simulink model "AWES3_CL_wTether_v4_PM"  (R2022a)
settings: Solver=ode3  StartTime=0  StopTime=simInit.TSIM  FixedStep=simInit.dt  RelTol=1e-3
values from neighbouring files (symbols this model uses):
  complex_tether_flag = 1    [run_sim.m]
  Ft_max = 1870    [run_sim.m]
  q = 0    [barrier_optimization.m]
  r = 0    [barrier_optimization.m]
  random_seed = [ 24335       17059       17670        1747]    [run_sim.m]
  safety_controller = false    [run_sim.m]
  turbulence = true    [run_sim.m]
undefined symbols (not defined in the file or in its folder): aeroModel, alpha_max, alpha_min, alpha_options, base_windspeed, constr, DiscIntNeverNeededParam, dx, ENVMT, F, grid_max, grid_min, HDBK, I_table, Light, MIL, mu_max, mu_min, mu_options, P_AP2, params, SampleTime, simInit, T, u0_sim, winchParameter, x0_sim
libraries: simulink x30, aerolibwind2 x14, dspstat3 x2, pid_lib x1, aerolibwindfilters x1, aerolibcommonsys x1, matrix_library x1
(part 1 of 5)
settings Model: SimulationMode=accelerator  ExtModeTrigDuration=100  Creator=Sebastian  LastModifiedBy=kebl6571
settings SolverCC: AlgebraicLoopSolver=LineSearch  DecoupledContinuousIntegration=on  MinimalZcImpactIntegration=on
settings DataIOCC: SaveFormat=StructureWithTime  SaveOutput=off  DSMLogging=off  SaveTime=off  StateSaveName=tmp_raccel_xout  OutputSaveName=logged_signals  SignalLoggingName=logged_signals  LoggingToFile=on  LoggingFileName=log.mat
settings OptimizationCC: BufferReuse=off  GlobalBufferReuse=off  ExpressionFolding=off  LocalBlockOutputs=off  EfficientMapNaN2IntZero=off  LifeSpan=inf  OptimizeDataStoreBuffers=off  BusAssignmentInplaceUpdate=off
settings DebuggingCC: ReadBeforeWriteMsg=DisableAll  WriteAfterWriteMsg=DisableAll  WriteAfterReadMsg=DisableAll  ArtificialAlgebraicLoopMsg=none  SaveWithDisabledLinksMsg=none  SaveWithParameterizedLinksMsg=none  MaskedZcDiagnostic=none  IgnoredZcDiagnostic=none  InheritedTsInSrcMsg=none  MultiTaskDSMMsg=none  TasksWithSamePriorityMsg=none  SigSpecEnsureSampleTimeMsg=none  BusObjectLabelMismatch=none  RootOutportRequireBusObject=none  AllowSymbolicDim=off  UnknownTsInhSupMsg=none  ModelReferenceDataLoggingMessage=none  ModelReferenceSymbolNameMessage=none  OperatingPointInterfaceChecksumMismatchMsg=none  InitInArrayFormatMsg=none  SFUnusedDataAndEventsDiag=none  SFUnexpectedBacktrackingDiag=none  SFInvalidInputDataAccessInChartInitDiag=none  SFNoUnconditionalDefaultTransitionDiag=none  SFTransitionOutsideNaturalParentDiag=none  SFUnreachableExecutionPathDiag=none  SFUndirectedBroadcastEventsDiag=none  SFTransitionActionBeforeConditionDiag=none  SFTemporalDelaySmallerThanSampleTimeDiag=none  SFSelfTransitionDiag=none  SFExecutionAtInitializationDiag=none  SFMachineParentedDataDiag=none  UnitsInconsistencyMsg=none  ArithmeticOperatorsInVariantConditions=warning
settings HardwareCC: TargetBitPerPointer=64  TargetBitPerSizeT=64  TargetBitPerPtrDiffT=64  TargetLongLongMode=on  TargetIntDivRoundTo=Zero  TargetEndianess=LittleEndian  TargetWordSize=64  TargetHWDeviceType=MATLAB Host  ProdEqTarget=off
settings ModelReferenceCC: UpdateModelReferenceTargets=IfOutOfDate  PropagateSignalLabelsOutOfModel=off
settings SFSimCC: SFSimEcho=off  SimUseLocalCustomCode=off  CustomCodeUndefinedFunction=UseInterfaceOnly
settings RTWCC: DLArmComputeVersion=19.05
settings CodeAppCC: MaxIdLength=128
settings GRTTargetCC: TargetLangStandard=C89/C90 (ANSI)  CombineOutputUpdateFcns=off  GRTInterface=on
settings ConfigComp: CovMetricSettings=dw  CovSaveCumulativeToWorkspaceVar=on  CovSaveSingleToWorkspaceVar=on  CovExternalEMLEnable=off

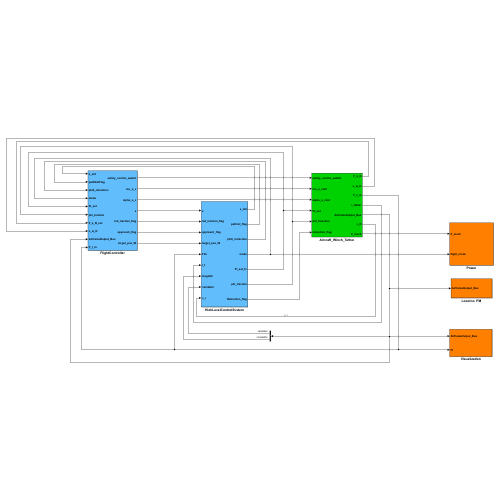
[thumbnail: Simulink's stored preview of the top-level diagram]
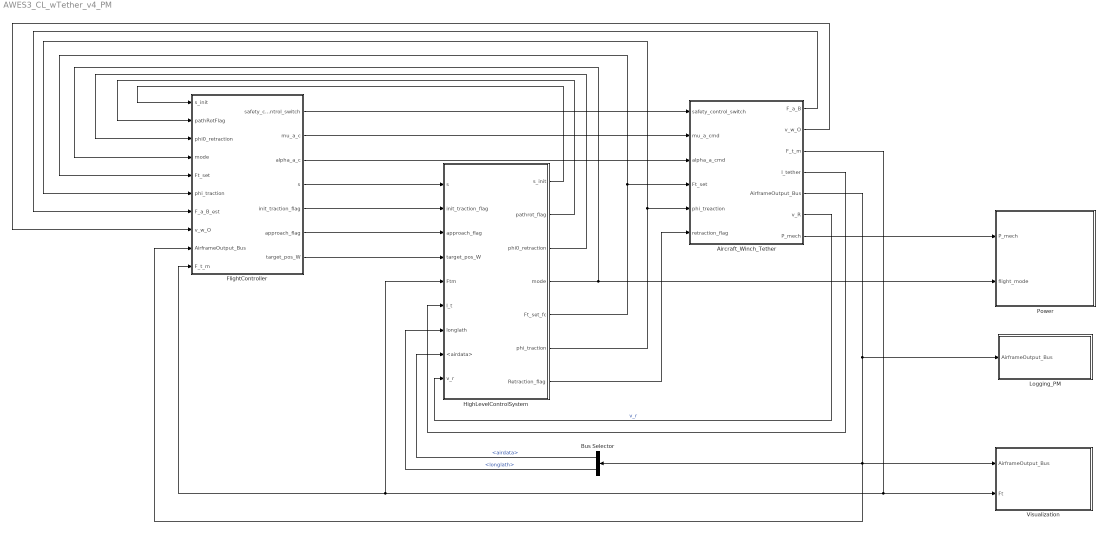
== system AWES3_CL_wTether_v4_PM ==
  Aircraft_Winch_Tether : Subsystem
  Bus Selector : BusSelector  OutputSignals=airdata,longlath
  FlightController : Subsystem
  HighLevelControlSystem : Subsystem
  Logging_PM : Subsystem  mask{logging_ts=0.01}
  Power : Subsystem  mask{sample_time=simInit.Ts_power_conv_check, min_cycles=4}
  Visualization : Subsystem
  wires:
  Aircraft_Winch_Tether/4(l_tether) -> HighLevelControlSystem/6(l_t)
  Aircraft_Winch_Tether/3(F_t_m) -> HighLevelControlSystem/5(Ftm), FlightController/10(F_t_m), Visualization/2(Ft)
  Aircraft_Winch_Tether/5(AirframeOutput_Bus) -> Visualization/1(AirframeOutput_Bus), FlightController/9(AirframeOutput_Bus), Bus Selector/1, Logging_PM/1(AirframeOutput_Bus)
  Bus Selector/2 -> HighLevelControlSystem/7(longlath)  "<longlath>"
  Aircraft_Winch_Tether/1(F_a_B) -> FlightController/7(F_a_B_est)
  Aircraft_Winch_Tether/2(v_w_O) -> FlightController/8(v_w_O)
  HighLevelControlSystem/4(mode) -> FlightController/4(mode), Power/2(flight_mode)
  HighLevelControlSystem/3(phi0_retraction) -> FlightController/3(phi0_retraction)
  HighLevelControlSystem/2(pathrot_flag) -> FlightController/2(pathRotFlag)
  HighLevelControlSystem/1(s_init) -> FlightController/1(s_init)
  HighLevelControlSystem/6(phi_traction) -> Aircraft_Winch_Tether/5(phi_treaction), FlightController/6(phi_traction)
  FlightController/4(s) -> HighLevelControlSystem/1(s)
  FlightController/5(init_traction_flag) -> HighLevelControlSystem/2(init_traction_flag)
  FlightController/6(approach_flag) -> HighLevelControlSystem/3(approach_flag)
  FlightController/7(target_pos_W) -> HighLevelControlSystem/4(target_pos_W)
  HighLevelControlSystem/5(Ft_set_fc) -> Aircraft_Winch_Tether/4(Ft_set), FlightController/5(Ft_set)
  HighLevelControlSystem/7(Retraction_flag) -> Aircraft_Winch_Tether/6(retraction_flag)
  Aircraft_Winch_Tether/6(v_R) -> HighLevelControlSystem/9(v_r)  "v_r"
  Bus Selector/1 -> HighLevelControlSystem/8(<airdata>)  "<airdata>"
  FlightController/3(alpha_a_c) -> Aircraft_Winch_Tether/3(alpha_a_cmd)
  FlightController/2(mu_a_c) -> Aircraft_Winch_Tether/2(mu_a_cmd)
  FlightController/1(safety_control_switch) -> Aircraft_Winch_Tether/1(safety_control_switch)
  Aircraft_Winch_Tether/7(P_mech) -> Power/1(P_mech)

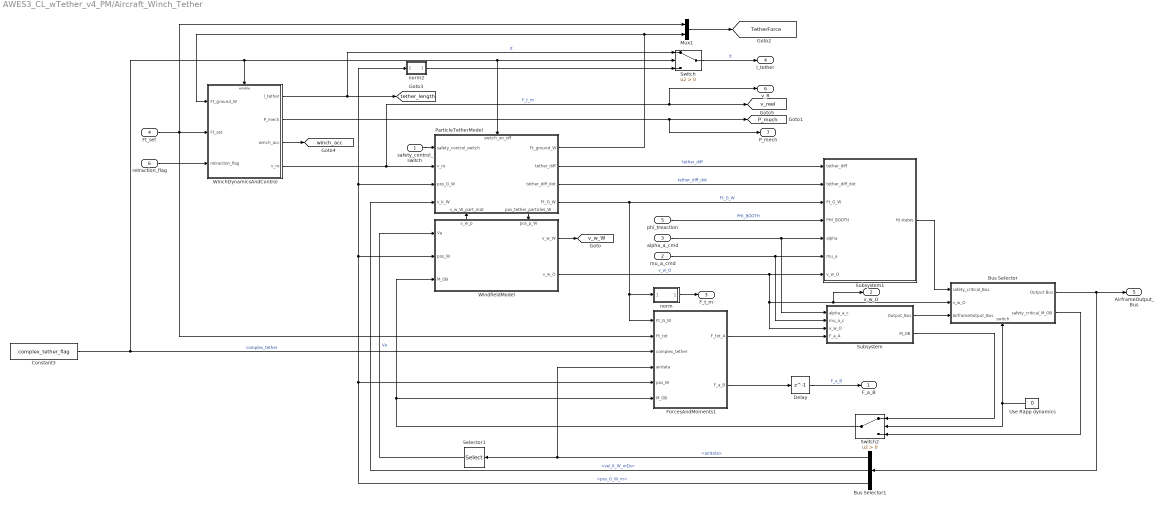
== system AWES3_CL_wTether_v4_PM/Aircraft_Winch_Tether ==
  safety_control_switch : Inport
  mu_a_cmd : Inport  Port=2  PortDimensions=1
  alpha_a_cmd : Inport  Port=3  PortDimensions=1
  Ft_set : Inport  Port=4  PortDimensions=1
  phi_treaction : Inport  Port=5  PortDimensions=1
  retraction_flag : Inport  Port=6  PortDimensions=1
  Bus Selector1 : BusSelector  OutputSignals=airdata,vel_K_W_mDs,pos_G_W_m
  Bus Selector : Subsystem
      settings: PortSchema="{\"entries\":[{\"content\":{\"sides\":[{\"content\":{\"connectorIds\":[\"In1\",\"In2\",\"In3\"]},\"type\":\"ConnectorPlacement.EquallySpacedRectSide\",\"uuid\":\"e2ab3ba8-f9f5-4bb0-af4c-3fe158d9c7f2\"},{\"content\":{\"connectorIds\":[\"Out1\",\"Out2\"],\"side\":\"RIGHT\"},\"type\":\"ConnectorPlacement.EquallySpacedRectSide\",\"uuid\":\"54795f1d-c357-49f1-9330-7dd1b9d78901\"},{\"content\":{\"connectorIds\":[],\"side\":\"TOP\"},\"type\":\"ConnectorPlacement.EquallySpacedRectSide\",\"uuid\":\"9cb9c5b8-3137-45d1-bfe3-c0a6ae4a4824\"},{\"content\":{\"connectorIds\":[\"In4\"],\"side\":\"BOTTOM\"},\"type\":\"ConnectorPlacement.EquallySpacedRectSide\",\"uuid\":\"b9adb0a8-6fab-4e9c-b487-f47b7669de1a\"}]},\"type\":\"ConnectorPlacement.EquallySpacedConnector\",\"uuid\":\"c66c7c14-26bf-43dc-ba87-485e61b07403\"}],\"packageUris\":[\"http://schema.mathworks.com/mf0/Connector/R2020b\"],\"version\":\"1.0\"}"
  Constant3 : Constant  Value=complex_tether_flag
  Delay : Delay  DelayLength=1  InitialCondition=[1;1;-P_AP2.mass*10]
  ForcesAndMoments1 : Subsystem
  Mux1 : Mux  Inputs=2
  ParticleTetherModel : Subsystem
      settings: PortSchema="{\"entries\":[{\"content\":{\"sides\":[{\"content\":{\"connectorIds\":[\"In1\",\"In2\",\"In3\",\"In4\"]},\"type\":\"ConnectorPlacement.EquallySpacedRectSide\",\"uuid\":\"ca78405c-c6d3-477d-b0a8-668910473732\"},{\"content\":{\"connectorIds\":[\"Out1\",\"Out2\",\"Out3\",\"Out4\"],\"side\":\"RIGHT\"},\"type\":\"ConnectorPlacement.EquallySpacedRectSide\",\"uuid\":\"a5c38c1a-07d2-4efb-bc49-b1eee8e8eb74\"},{\"content\":{\"connectorIds\":[\"In5\"],\"side\":\"TOP\"},\"type\":\"ConnectorPlacement.EquallySpacedRectSide\",\"uuid\":\"403c634d-ac4b-4d6b-b076-489af818e83e\"},{\"content\":{\"connectorIds\":[\"In6\",\"Out5\"],\"side\":\"BOTTOM\"},\"type\":\"ConnectorPlacement.EquallySpacedRectSide\",\"uuid\":\"4ef9c4e3-0026-4b23-9119-1a1dd44b231c\"}]},\"type\":\"ConnectorPlacement.EquallySpacedConnector\",\"uuid\":\"599465da-399f-49af-adc9-4f96ef4c12cd\"}],\"packageUris\":[\"http://schema.mathworks.com/mf0/Connector/R2020b\"],\"version\":\"1.0\"}"
  Selector1 : Selector  InputPortWidth=3  IndexOptions=Index vector (dialog)  Indices=1  OutputSizes=1
  Subsystem : Subsystem
      settings: MinAlgLoopOccurrences=on
  Subsystem1 : Subsystem
      settings: MinAlgLoopOccurrences=on
  Switch : Switch  Criteria=u2 > Threshold  SaturateOnIntegerOverflow=off  InputSameDT=off
  Switch2 : Switch  Criteria=u2 > Threshold  SaturateOnIntegerOverflow=off  InputSameDT=off
  Use Rapp dynamics : Constant  Value=0
  "WinchDynamicsAndControl " : Subsystem
  WindfieldModel : Subsystem  TreatAsAtomicUnit=on
      settings: MinAlgLoopOccurrences=on  PortSchema="{\"entries\":[{\"content\":{\"sides\":[{\"content\":{\"connectorIds\":[\"In1\",\"In2\",\"In3\"]},\"type\":\"ConnectorPlacement.EquallySpacedRectSide\",\"uuid\":\"5214d961-fdb0-4544-8128-59e00c6649fb\"},{\"content\":{\"connectorIds\":[\"Out1\",\"Out2\"],\"side\":\"RIGHT\"},\"type\":\"ConnectorPlacement.EquallySpacedRectSide\",\"uuid\":\"cdd5f5d4-5bc0-4393-ba09-7e71cbb012db\"},{\"content\":{\"connectorIds\":[\"Out3\",\"In4\"],\"side\":\"TOP\"},\"type\":\"ConnectorPlacement.EquallySpacedRectSide\",\"uuid\":\"608e5071-fd31-4d22-8974-ba91486c9a41\"}]},\"type\":\"ConnectorPlacement.EquallySpacedConnector\",\"uuid\":\"a45b9672-4292-4679-90b4-f0e0bc01633b\"}],\"packageUris\":[\"http://schema.mathworks.com/mf0/Connector/R2020b\"],\"version\":\"1.0\"}"
  norm : Subsystem
  norm2 : Subsystem
  F_a_B : Outport  VectorParamsAs1DForOutWhenUnconnected=off
  v_w_O : Outport  Port=2  VectorParamsAs1DForOutWhenUnconnected=off
  F_t_m : Outport  Port=3  VectorParamsAs1DForOutWhenUnconnected=off
  l_tether : Outport  Port=4  VectorParamsAs1DForOutWhenUnconnected=off
  AirframeOutput_Bus : Outport  Port=5  VectorParamsAs1DForOutWhenUnconnected=off
  v_R : Outport  Port=6  VectorParamsAs1DForOutWhenUnconnected=off
  P_mech : Outport  Port=7  VectorParamsAs1DForOutWhenUnconnected=off
  tag scope: P_mech=global, TetherForce=global, tether_length=global, v_reel=global, v_w_W=global, winch_acc=global
  wires:
  ForcesAndMoments1/2(F_a_B) -> Delay/1
  WindfieldModel/1(v_w_W) -> [v_w_W]
  WindfieldModel/3(v_w_p) -> ParticleTetherModel/6(v_w_W_part_mat)
  ParticleTetherModel/1(Ft_ground_W) -> Mux1/2, "WinchDynamicsAndControl "/1(Ft_ground_W)
  Ft_set/1 -> "WinchDynamicsAndControl "/2(Ft_set), Mux1/1, ForcesAndMoments1/2(Ft_tot)
  ParticleTetherModel/5(pos_tether_particles_W) -> WindfieldModel/4(pos_p_W)
  Delay/1 -> F_a_B/1  "F_a_B"
  WindfieldModel/2(v_w_O) -> Bus Selector/2(v_w_O), v_w_O/1, Subsystem/3(v_w_O), Subsystem1/7(v_w_O)  "v_w_O"
  Switch/1 -> l_tether/1  "lt"
  ParticleTetherModel/4(Ft_G_W) -> norm/1(Ft_G_W), ForcesAndMoments1/1(Ft_G_W), Subsystem1/3(Ft_G_W)  "Ft_G_W"
  "WinchDynamicsAndControl "/4(v_ro) -> ParticleTetherModel/2(v_ro), v_R/1, [v_reel]  "F_t_m"
  Constant3/1 -> ParticleTetherModel/5(switch_on_off), Switch/2, "WinchDynamicsAndControl "/Enable, ForcesAndMoments1/3(complex_tether)  "complex_tether"
  mu_a_cmd/1 -> Subsystem/2(mu_a_c), Subsystem1/6(mu_a)
  Switch2/1 -> ForcesAndMoments1/6(M_OB), WindfieldModel/3(M_OB)
  "WinchDynamicsAndControl "/3(winch_acc) -> [winch_acc]
  "WinchDynamicsAndControl "/2(P_mech) -> P_mech/1, [P_mech]
  Mux1/1 -> [TetherForce]
  "WinchDynamicsAndControl "/1(l_tether) -> [tether_length], Switch/1  "lt"
  alpha_a_cmd/1 -> Subsystem/1(alpha_a_c), Subsystem1/5(alpha)
  Bus Selector1/2 -> ParticleTetherModel/4(v_k_W)  "<vel_K_W_mDs>"
  Bus Selector1/3 -> ForcesAndMoments1/5(pos_W), ParticleTetherModel/3(pos_G_W), norm2/1(<pos_G_W_m>), WindfieldModel/2(pos_W)  "<pos_G_W_m>"
  Bus Selector/2(safety_critical_M_OB) -> Switch2/3
  Bus Selector1/1 -> Selector1/1, ForcesAndMoments1/4(airdata)  "<airdata>"
  Selector1/1 -> WindfieldModel/1(Va)  "Va"
  Use Rapp dynamics/1 -> Switch2/2, Bus Selector/4(switch)
  retraction_flag/1 -> "WinchDynamicsAndControl "/3(retraction_flag)
  safety_control_switch/1 -> ParticleTetherModel/1(safety_control_switch)
  Subsystem1/1(HJ states) -> Bus Selector/1(safety_critical_Bus)
  ParticleTetherModel/2(tether_diff) -> Subsystem1/1(tether_diff)  "tether_diff"
  ParticleTetherModel/3(tether_diff_dot) -> Subsystem1/2(tether_diff_dot)  "tether_diff_dot"
  phi_treaction/1 -> Subsystem1/4(PHI_BOOTH)  "PHI_BOOTH"
  ForcesAndMoments1/1(F_tot_A) -> Subsystem/4(F_a_A)
  Subsystem/2(M_OB) -> Switch2/1
  Subsystem/1(Output_Bus) -> Bus Selector/3(AirframeOutput_Bus)
  norm/1(F_t_m) -> F_t_m/1
  norm2/1(Out1) -> Switch/3
  Bus Selector/1(Output Bus) -> Bus Selector1/1, AirframeOutput_Bus/1

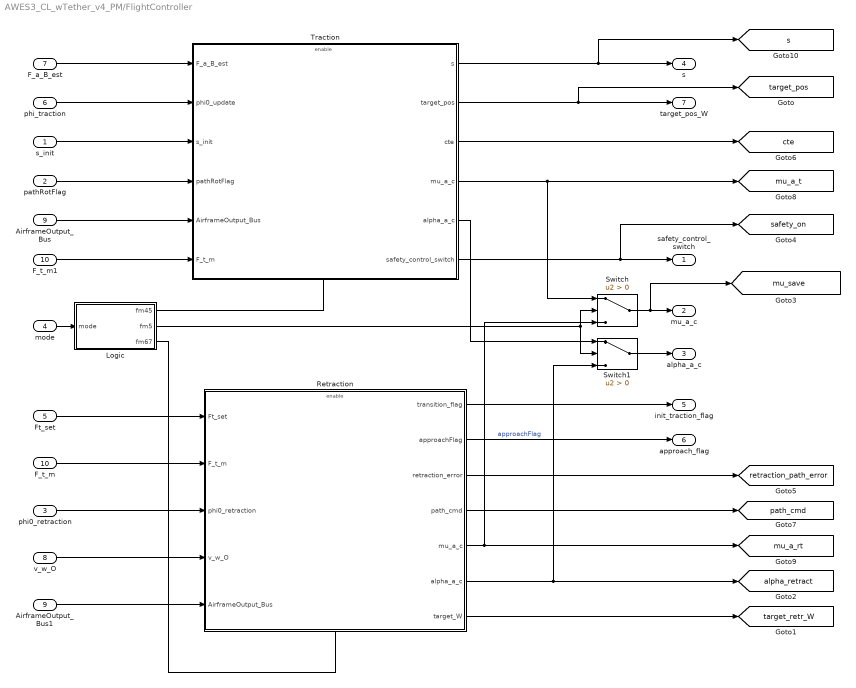
== system AWES3_CL_wTether_v4_PM/FlightController ==
  s_init : Inport
  pathRotFlag : Inport  Port=2
  phi0_retraction : Inport  Port=3
  mode : Inport  Port=4
  Ft_set : Inport  Port=5
  phi_traction : Inport  Port=6
  F_a_B_est : Inport  Port=7
  v_w_O : Inport  Port=8
  AirframeOutput_Bus : Inport  Port=9
  F_t_m : Inport  Port=10
  AirframeOutput_Bus1 : InportShadow  Port=9
  F_t_m1 : InportShadow  Port=10
  Logic : Subsystem
  Retraction : Subsystem
  Switch : Switch  Criteria=u2 > Threshold  SaturateOnIntegerOverflow=off  InputSameDT=off
  Switch1 : Switch  Criteria=u2 > Threshold  SaturateOnIntegerOverflow=off  InputSameDT=off
  Traction : Subsystem
  safety_control_switch : Outport
  mu_a_c : Outport  Port=2  VectorParamsAs1DForOutWhenUnconnected=off
  alpha_a_c : Outport  Port=3  VectorParamsAs1DForOutWhenUnconnected=off
  s : Outport  Port=4  VectorParamsAs1DForOutWhenUnconnected=off
  init_traction_flag : Outport  Port=5  VectorParamsAs1DForOutWhenUnconnected=off
  approach_flag : Outport  Port=6  VectorParamsAs1DForOutWhenUnconnected=off
  target_pos_W : Outport  Port=7  VectorParamsAs1DForOutWhenUnconnected=off
  tag scope: alpha_retract=global, cte=global, mu_a_rt=global, mu_a_t=global, mu_save=global, path_cmd=global, retraction_path_error=global, s=global, safety_on=global, target_pos=global, target_retr_W=global
  wires:
  F_a_B_est/1 -> Traction/1(F_a_B_est)
  phi_traction/1 -> Traction/2(phi0_update)
  s_init/1 -> Traction/3(s_init)
  pathRotFlag/1 -> Traction/4(pathRotFlag)
  Ft_set/1 -> Retraction/1(Ft_set)
  F_t_m/1 -> Retraction/2(F_t_m)
  phi0_retraction/1 -> Retraction/3(phi0_retraction)
  v_w_O/1 -> Retraction/4(v_w_O)
  mode/1 -> Logic/1(mode)
  Logic/1(fm45) -> Traction/Enable
  Logic/2(fm5) -> Switch1/2, Switch/2
  Logic/3(fm67) -> Retraction/Enable
  Retraction/5(mu_a_c) -> [mu_a_rt], Switch/3
  Switch/1 -> [mu_save], mu_a_c/1
  Retraction/1(transition_flag) -> init_traction_flag/1
  Retraction/2(approachFlag) -> approach_flag/1  "approachFlag"
  Traction/2(target_pos) -> [target_pos], target_pos_W/1
  Traction/1(s) -> s/1, [s]
  AirframeOutput_Bus/1 -> Traction/5(AirframeOutput_Bus)
  AirframeOutput_Bus1/1 -> Retraction/5(AirframeOutput_Bus)
  Retraction/6(alpha_a_c) -> Switch1/3, [alpha_retract]
  Retraction/3(retraction_error) -> [retraction_path_error]
  Traction/3(cte) -> [cte]
  Retraction/4(path_cmd) -> [path_cmd]
  Traction/4(mu_a_c) -> Switch/1, [mu_a_t]
  Switch1/1 -> alpha_a_c/1
  Traction/5(alpha_a_c) -> Switch1/1
  Retraction/7(target_W) -> [target_retr_W]
  Traction/6(safety_control_switch) -> [safety_on], safety_control_switch/1
  F_t_m1/1 -> Traction/6(F_t_m)

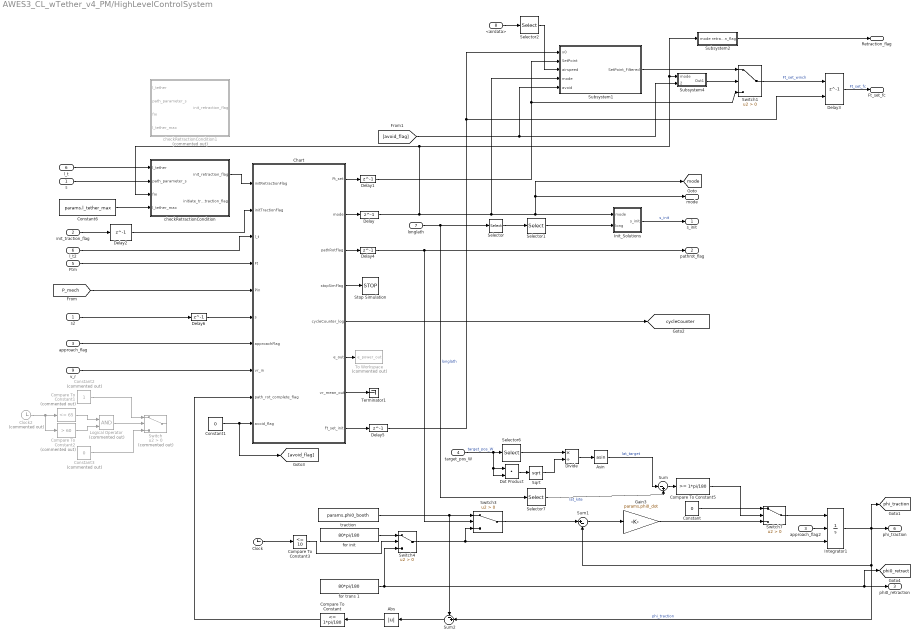
== system AWES3_CL_wTether_v4_PM/HighLevelControlSystem ==
  s : Inport
  init_traction_flag : Inport  Port=2
  approach_flag : Inport  Port=3
  target_pos_W : Inport  Port=4
  Ftm : Inport  Port=5
  l_t : Inport  Port=6
  longlath : Inport  Port=7
  <airdata> : Inport  Port=8
  v_r : Inport  Port=9
  Abs : Abs  SaturateOnIntegerOverflow=off
  Asin : Trigonometry  Operator=asin
  Chart : Stateflow chart  TreatAsAtomicUnit=on  mask{Ft_set_traction=params.Ft_set_traction, Ft_set_traction_low=params.Ft_set_traction_low, Ft_set_retraction=params.Ft_set_retraction, l_t_min_max=params.l_t_min_max, cycleCounterMin=3, cycleCounterMax=5, e_conv=constr.F_t_max*constr.winchParameter.v_max*0.001, Vamin=constr.vamin, vr_mean_min=params.vr_mean_min, Ft_set_avoidance=1200, trac_count_max=10}
  Clock : Clock
  Clock2 : Clock  Commented=on
  Compare To Constant : simulink/Logic and Bit Operations/Compare To Constant  relop=<=  const=1*pi/180  OutDataTypeStr=boolean
  Compare To Constant1 : simulink/Logic and Bit Operations/Compare To Constant  Commented=on  relop=<=  const=65  OutDataTypeStr=boolean
  Compare To Constant2 : simulink/Logic and Bit Operations/Compare To Constant  Commented=on  relop=>  const=60  OutDataTypeStr=boolean
  Compare To Constant3 : simulink/Logic and Bit Operations/Compare To Constant  relop=<=  const=10  OutDataTypeStr=boolean
  Compare To Constant5 : simulink/Logic and Bit Operations/Compare To Constant  relop=>=  const=1*pi/180  OutDataTypeStr=boolean
  Constant : Constant  Value=0
  Constant1 : Constant  Value=0
  Constant2 : Constant  Commented=on
  Constant3 : Constant  Commented=on  Value=0
  Constant6 : Constant  Value=params.l_tether_max
  Delay : Delay  DelayLength=1  InitialCondition=5
  Delay1 : Delay  DelayLength=1  InitialCondition=100
  Delay2 : Delay  DelayLength=1  InitialCondition=5
  Delay3 : Delay  DelayLength=1  InitialConditionSource=Input port  InitialCondition=500
      settings: InputPortMap=u0,p4
  Delay4 : Delay  DelayLength=1
  Delay5 : Delay  DelayLength=1  InitialCondition=1000
  Delay6 : Delay  DelayLength=1  InitialCondition=0
  Divide : Product  Inputs=*/
  Dot Product : DotProduct  OutDataTypeStr=Inherit: Inherit via internal rule
  Gain3 : Gain  Gain=params.phi0_dot
  Init_Solutions : Stateflow chart  TreatAsAtomicUnit=on
  Integrator1 : Integrator  ExternalReset=rising  InitialConditionSource=external
  Logical Operator : Logic  Commented=on  AllPortsSameDT=off  OutDataTypeStr=boolean
  Selector : Selector  InputPortWidth=3  IndexOptions=Index vector (dialog)  Indices=1:2  OutputSizes=1
  Selector1 : Selector  InputPortWidth=2  IndexOptions=Index vector (dialog)  Indices=1  OutputSizes=1
  Selector2 : Selector  InputPortWidth=3  IndexOptions=Index vector (dialog)  Indices=1  OutputSizes=1
  Selector6 : Selector  InputPortWidth=3  IndexOptions=Index vector (dialog)  Indices=3  OutputSizes=1
  Selector7 : Selector  InputPortWidth=3  IndexOptions=Index vector (dialog)  Indices=2  OutputSizes=1
  Sqrt : Sqrt
  Stop Simulation : Stop
  Subsystem1 : Subsystem  mask{w0=0.25}
  Subsystem2 : Subsystem
  Subsystem4 : Subsystem
  Sum : Sum  Inputs=|-+
  Sum1 : Sum  Inputs=|+-
  Sum2 : Sum  Inputs=-+|
  Switch : Switch  Commented=on  Criteria=u2 > Threshold  SaturateOnIntegerOverflow=off  InputSameDT=off
  Switch{1,3..4,7} (4 alike) : Switch  Criteria=u2 > Threshold  SaturateOnIntegerOverflow=off  InputSameDT=off
  Terminator1 : Terminator
  To Workspace : ToWorkspace  Commented=on  VariableName=e_power_out  SaveFormat=Timeseries  SampleTime=0.1
  approach_flag2 : InportShadow  Port=3
  checkRetractionCondition : Stateflow chart  TreatAsAtomicUnit=on  mask{delta_s_1=params.eject2retraction-pi/180, delta_s_2=params.eject2retraction}
  checkRetractionCondition1 : Stateflow chart  Commented=on  TreatAsAtomicUnit=on  mask{delta_s_1=29*pi/180, delta_s_2=30*pi/180}
  for init : Constant  Value=80*pi/180
  for trans 1 : Constant  Value=80*pi/180
  l_t2 : InportShadow  Port=6
  s2 : InportShadow
  traction : Constant  Value=params.phi0_booth
  s_init : Outport  VectorParamsAs1DForOutWhenUnconnected=off
  pathrot_flag : Outport  Port=2  VectorParamsAs1DForOutWhenUnconnected=off
  phi0_retraction : Outport  Port=3  VectorParamsAs1DForOutWhenUnconnected=off
  mode : Outport  Port=4  VectorParamsAs1DForOutWhenUnconnected=off
  Ft_set_fc : Outport  Port=5  PortDimensions=1  VectorParamsAs1DForOutWhenUnconnected=off
  phi_traction : Outport  Port=6  VectorParamsAs1DForOutWhenUnconnected=off
  Retraction_flag : Outport  Port=7  VectorParamsAs1DForOutWhenUnconnected=off
  tag scope: cycleCounter=global, mode=global, phi0_retract=global, phi_traction=global
  wires:
  Subsystem1/1(SetPoint_Filtered) -> Switch1/1
  [P_mech] -> Chart/5(Pin)
  Chart/4(stopSimFlag) -> Stop Simulation/1
  Chart/3(pathRotFlag) -> Delay4/1
  Selector1/1 -> Init_Solutions/2(long)
  Delay1/1 -> Subsystem1/2(SetPoint), Switch1/3
  Compare To Constant3/1 -> Switch4/2
  for trans 1/1 -> [phi0_retract], phi0_retraction/1, Switch4/3
  Chart/5(cycleCounter_log) -> [cycleCounter]
  Delay/1 -> Init_Solutions/1(mode), [mode], mode/1, Subsystem1/4(mode), checkRetractionCondition/3(fm), Subsystem2/1(mode), Subsystem4/1(mode)
  Ftm/1 -> Chart/4(Ft)
  Constant6/1 -> checkRetractionCondition/4(l_tether_max)
  Delay3/1 -> Ft_set_fc/1  "Ft_set_fc"
  checkRetractionCondition/1(init_retraction_flag) -> Chart/1(initRetractionFlag)
  Switch1/1 -> Delay3/1  "Ft_set_winch"
  Chart/1(Ft_set) -> Delay1/1
  approach_flag/1 -> Chart/7(approachFlag)
  Chart/2(mode) -> Delay/1
  traction/1 -> Switch3/1, Sum2/1
  for init/1 -> Switch4/1
  Clock/1 -> Compare To Constant3/1
  l_t2/1 -> Chart/3(l_t)
  s/1 -> checkRetractionCondition/2(path_parameter_s)
  init_traction_flag/1 -> Delay2/1
  Selector/1 -> Selector1/1
  l_t/1 -> checkRetractionCondition/1(l_tether)
  Chart/8(Ft_set_init) -> Delay5/1
  Delay4/1 -> Switch3/2, pathrot_flag/1
  Delay2/1 -> Chart/2(initTractionFlag)
  longlath/1 -> Selector7/1, Selector/1  "longlath"
  Divide/1 -> Asin/1
  target_pos_W/1 -> Dot Product/2, Dot Product/1, Selector6/1  "target_pos_W"
  Selector7/1 -> Sum/2  "lat_kite"
  Selector6/1 -> Divide/1
  Dot Product/1 -> Sqrt/1
  Sum/1 -> Compare To Constant5/1
  Asin/1 -> Sum/1  "lat_target"
  Sqrt/1 -> Divide/2
  Compare To Constant5/1 -> Switch7/2
  Constant/1 -> Switch7/1
  Gain3/1 -> Switch7/3
  Switch3/1 -> Sum1/1
  Switch7/1 -> Integrator1/1
  Sum1/1 -> Gain3/1
  Switch4/1 -> Integrator1/3, Switch3/3
  approach_flag2/1 -> Integrator1/2
  Subsystem2/1(retraction_flag) -> Retraction_flag/1
  Chart/6(e_out) -> To Workspace/1
  Sum2/1 -> Abs/1
  Abs/1 -> Compare To Constant/1
  Compare To Constant/1 -> Chart/9(path_rot_complete_flag)
  v_r/1 -> Chart/8(vr_in)
  Chart/7(vr_mean_out) -> Terminator1/1
  Integrator1/1 -> Sum1/2, Sum2/2, phi_traction/1, [phi_traction]  "phi_traction"
  <airdata>/1 -> Selector2/1
  Selector2/1 -> Subsystem1/3(airspeed)
  Constant2/1 -> Switch/1
  Constant3/1 -> Switch/3
  Clock2/1 -> Compare To Constant2/1, Compare To Constant1/1
  Compare To Constant1/1 -> Logical Operator/1
  Logical Operator/1 -> Switch/2
  Compare To Constant2/1 -> Logical Operator/2
  [avoid_flag] -> Subsystem1/5(avoid), Subsystem4/2(avoid_flag)
  Delay5/1 -> Subsystem1/1(x0), Delay3/2
  Subsystem4/1(Out1) -> Switch1/2
  Constant1/1 -> [avoid_flag], Chart/10(avoid_flag)
  Init_Solutions/1(s_init) -> s_init/1  "s_init"
  Delay6/1 -> Chart/6(s)
  s2/1 -> Delay6/1

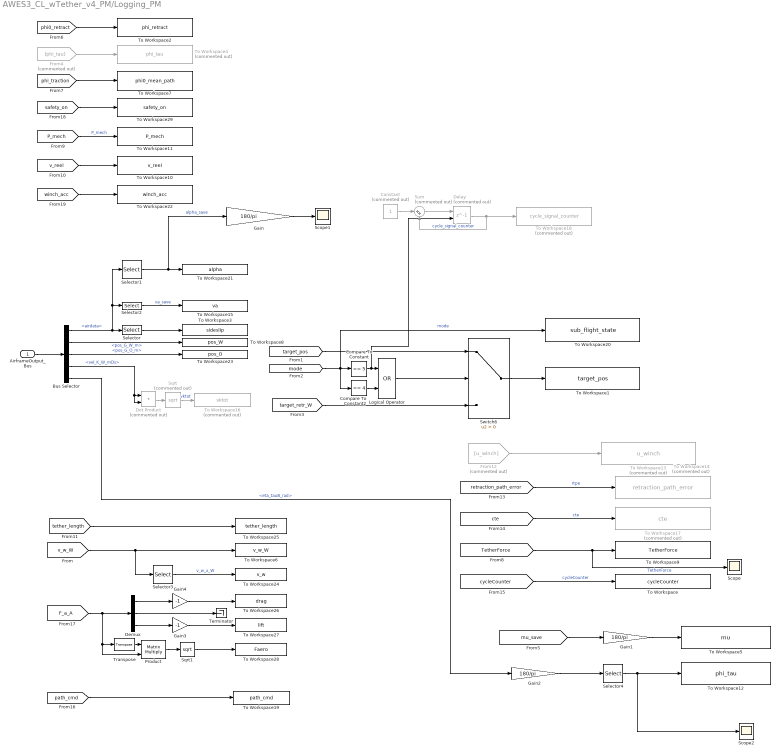
== system AWES3_CL_wTether_v4_PM/Logging_PM ==
  AirframeOutput_Bus : Inport
  Bus Selector : BusSelector  OutputSignals=airdata,pos_G_W_m,pos_G_O_m,vel_K_W_mDs,eta_tauB_rad
  Compare To Constant : simulink/Logic and Bit Operations/Compare To Constant  relop===  const=5  OutDataTypeStr=boolean
  Compare To Constant2 : simulink/Logic and Bit Operations/Compare To Constant  relop===  const=4  OutDataTypeStr=boolean
  Constant : Constant  Commented=on
  Delay : Delay  Commented=on  DelayLength=1  ExternalReset=Rising  SampleTime=logging_ts
      settings: InputPortMap=u0,r5
  Demux : Demux  Outputs=3
  Dot Product : DotProduct  Commented=on  OutDataTypeStr=Inherit: Inherit via internal rule
  From12 : From  Commented=on  GotoTag=u_winch  TagVisibility=global
  From4 : From  Commented=on  GotoTag=phi_tau  TagVisibility=global
  Gain : Gain  Gain=180/pi
  Gain1 : Gain  Gain=180/pi
  Gain2 : Gain  Gain=180/pi
  Gain3 : Gain  Gain=-1
  Gain4 : Gain  Gain=-1
  Logical Operator : Logic  Operator=OR  AllPortsSameDT=off  OutDataTypeStr=boolean
  Product : Product  Multiplication=Matrix(*)
  Scope : Scope
  Scope1 : Scope
  Scope2 : Scope
  Selector : Selector  InputPortWidth=3  IndexOptions=Index vector (dialog)  Indices=3  OutputSizes=1
  Selector1 : Selector  InputPortWidth=3  IndexOptions=Index vector (dialog)  Indices=2  OutputSizes=1
  Selector2 : Selector  InputPortWidth=3  IndexOptions=Index vector (dialog)  Indices=1  OutputSizes=1
  Selector3 : Selector  InputPortWidth=3  IndexOptions=Index vector (dialog)  Indices=1  OutputSizes=1
  Selector4 : Selector  InputPortWidth=3  IndexOptions=Index vector (dialog)  Indices=1:2  OutputSizes=1
  Sqrt : Sqrt  Commented=on
  Sqrt1 : Sqrt
  Sum : Sum  Commented=on  Inputs=|++
  Switch6 : Switch  Criteria=u2 > Threshold  SaturateOnIntegerOverflow=off  InputSameDT=off
  Terminator : Terminator
  To Workspace : ToWorkspace  VariableName=cycleCounter  SaveFormat=Timeseries  SampleTime=-1
      settings: MaxDataPoints=1
  To Workspace1 : ToWorkspace  VariableName=target_pos  SaveFormat=Timeseries  SampleTime=logging_ts
  To Workspace10 : ToWorkspace  VariableName=v_reel  SaveFormat=Timeseries  SampleTime=logging_ts
  To Workspace11 : ToWorkspace  VariableName=P_mech  SaveFormat=Timeseries  SampleTime=logging_ts
  To Workspace12 : ToWorkspace  VariableName=phi_tau  SaveFormat=Timeseries  SampleTime=logging_ts
  To Workspace13 : ToWorkspace  Commented=on  VariableName=u_winch  SaveFormat=Timeseries  SampleTime=logging_ts
  To Workspace14 : ToWorkspace  Commented=on  VariableName=retraction_path_error  SaveFormat=Timeseries  SampleTime=logging_ts
  To Workspace15 : ToWorkspace  VariableName=va  SaveFormat=Timeseries  SampleTime=logging_ts
  To Workspace16 : ToWorkspace  Commented=on  VariableName=vktot  SaveFormat=Timeseries  SampleTime=logging_ts
  To Workspace17 : ToWorkspace  Commented=on  VariableName=cte  SaveFormat=Timeseries  SampleTime=logging_ts
  To Workspace18 : ToWorkspace  Commented=on  VariableName=cycle_signal_counter  SaveFormat=Timeseries  SampleTime=logging_ts
      settings: MaxDataPoints=1
  To Workspace19 : ToWorkspace  VariableName=path_cmd  SaveFormat=Timeseries  SampleTime=logging_ts
  To Workspace2 : ToWorkspace  VariableName=phi_retract  SaveFormat=Timeseries  SampleTime=logging_ts
  To Workspace20 : ToWorkspace  VariableName=sub_flight_state  SaveFormat=Timeseries  SampleTime=logging_ts
  To Workspace21 : ToWorkspace  VariableName=alpha  SaveFormat=Timeseries  SampleTime=logging_ts
  To Workspace22 : ToWorkspace  VariableName=winch_acc  SaveFormat=Timeseries  SampleTime=logging_ts
  To Workspace23 : ToWorkspace  VariableName=pos_O  SaveFormat=Timeseries  SampleTime=logging_ts
  To Workspace24 : ToWorkspace  VariableName=v_w  SaveFormat=Timeseries  SampleTime=logging_ts
  To Workspace25 : ToWorkspace  VariableName=tether_length  SaveFormat=Timeseries  SampleTime=logging_ts
  To Workspace26 : ToWorkspace  VariableName=drag  SaveFormat=Timeseries  SampleTime=logging_ts
  To Workspace27 : ToWorkspace  VariableName=lift  SaveFormat=Timeseries  SampleTime=logging_ts
  To Workspace28 : ToWorkspace  VariableName=Faero  SaveFormat=Timeseries  SampleTime=logging_ts
  To Workspace29 : ToWorkspace  VariableName=safety_on  SaveFormat=Timeseries  SampleTime=logging_ts
  To Workspace3 : ToWorkspace  VariableName=sideslip  SaveFormat=Timeseries  SampleTime=logging_ts
  To Workspace4 : ToWorkspace  Commented=on  VariableName=phi_tau  SaveFormat=Timeseries  SampleTime=logging_ts
  To Workspace5 : ToWorkspace  VariableName=mu  SaveFormat=Timeseries  SampleTime=logging_ts
  To Workspace6 : ToWorkspace  VariableName=v_w_W  SaveFormat=Timeseries  SampleTime=logging_ts
  To Workspace7 : ToWorkspace  VariableName=phi0_mean_path  SaveFormat=Timeseries  SampleTime=logging_ts
  To Workspace8 : ToWorkspace  VariableName=pos_W  SaveFormat=Timeseries  SampleTime=logging_ts
  To Workspace9 : ToWorkspace  VariableName=TetherForce  SaveFormat=Timeseries  SampleTime=logging_ts
  Transpose : matrix_library/Transpose
      settings: SourceProductBaseCode=SL
  wires:
  Switch6/1 -> To Workspace1/1
  [target_pos] -> Switch6/1
  Logical Operator/1 -> Switch6/2
  [target_retr_W] -> Switch6/3
  From4/1 -> To Workspace4/1
  [phi0_retract] -> To Workspace2/1
  [phi_traction] -> To Workspace7/1
  Selector/1 -> To Workspace3/1
  AirframeOutput_Bus/1 -> Bus Selector/1
  Bus Selector/1 -> Selector1/1, Selector2/1, Selector/1  "<airdata>"
  [v_w_W] -> Selector3/1, To Workspace6/1
  Bus Selector/2 -> To Workspace8/1  "<pos_G_W_m>"
  Compare To Constant/1 -> Delay/2, Logical Operator/1
  Compare To Constant2/1 -> Logical Operator/2
  [TetherForce] -> Scope/1, To Workspace9/1  "TetherForce"
  [v_reel] -> To Workspace10/1
  [P_mech] -> To Workspace11/1  "P_mech"
  From12/1 -> To Workspace13/1
  [retraction_path_error] -> To Workspace14/1  "rtpe"
  Selector2/1 -> To Workspace15/1  "va_save"
  Bus Selector/4 -> Dot Product/2, Dot Product/1  "<vel_K_W_mDs>"
  Dot Product/1 -> Sqrt/1
  Sqrt/1 -> To Workspace16/1  "vktot"
  [cte] -> To Workspace17/1  "cte"
  Selector3/1 -> To Workspace24/1  "v_w_x_W"
  Constant/1 -> Sum/1
  Sum/1 -> Delay/1
  Delay/1 -> To Workspace18/1, Sum/2  "cycle_signal_counter"
  [mode] -> To Workspace20/1, Compare To Constant2/1, Compare To Constant/1  "mode"
  [cycleCounter] -> To Workspace/1  "cycleCounter"
  [path_cmd] -> To Workspace19/1
  [winch_acc] -> To Workspace22/1
  Selector1/1 -> Gain/1, To Workspace21/1  "alpha_save"
  Gain/1 -> Scope1/1
  [mu_save] -> Gain1/1
  Gain1/1 -> To Workspace5/1
  Bus Selector/5 -> Gain2/1  "<eta_tauB_rad>"
  Gain2/1 -> Selector4/1
  Selector4/1 -> Scope2/1, To Workspace12/1
  Bus Selector/3 -> To Workspace23/1  "<pos_G_O_m>"
  [tether_length] -> To Workspace25/1
  [F_a_A] -> Transpose/1, Product/2, Demux/1
  Demux/3 -> Gain3/1
  Demux/1 -> Gain4/1
  Demux/2 -> Terminator/1
  Gain4/1 -> To Workspace26/1
  Gain3/1 -> To Workspace27/1
  Product/1 -> Sqrt1/1
  Sqrt1/1 -> To Workspace28/1
  [safety_on] -> To Workspace29/1
  Transpose/1 -> Product/1

== system AWES3_CL_wTether_v4_PM/Power ==
  P_mech : Inport
  flight_mode : Inport  Port=2
  Compare To Constant : simulink/Logic and Bit Operations/Compare To Constant  relop=>=  const=min_cycles  OutDataTypeStr=boolean
  Constant : Constant  Value=simInit.power_conv_threshold
  Delay{,1..6} (7 alike) : Delay  DelayLength=1  InitialCondition=0
  Logical Operator : Logic  AllPortsSameDT=off  OutDataTypeStr=boolean
  MATLAB Function : MATLAB Function  TreatAsAtomicUnit=on
  Rate Transition{,1..6} (7 alike) : RateTransition  OutPortSampleTime=sample_time
  Relational Operator : RelationalOperator  Operator=<=  OutDataTypeStr=boolean  RndMeth=Simplest  InputSameDT=off
  Stop Simulation : Stop
  To Workspace18 : ToWorkspace  VariableName=cycle_signal_counter  SaveFormat=Timeseries  SampleTime=-1
  wires:
  P_mech/1 -> Rate Transition/1
  Rate Transition/1 -> MATLAB Function/5(u)
  flight_mode/1 -> Rate Transition1/1
  Rate Transition1/1 -> MATLAB Function/6(flightMode)
  Delay/1 -> MATLAB Function/1("flag ")
  MATLAB Function/1(flag) -> Delay/1
  MATLAB Function/2(m_new) -> Rate Transition2/1
  MATLAB Function/3(p_sum) -> Rate Transition3/1
  MATLAB Function/4(cnt) -> Rate Transition4/1
  MATLAB Function/5(e_new) -> Rate Transition5/1
  MATLAB Function/6(cnt_max_mat) -> Rate Transition6/1
  Rate Transition2/1 -> Delay1/1
  Rate Transition3/1 -> Delay2/1
  Rate Transition4/1 -> Delay3/1
  Delay1/1 -> MATLAB Function/2(m_old)
  Delay2/1 -> MATLAB Function/3("p_sum ")
  Delay3/1 -> MATLAB Function/4("cnt ")
  MATLAB Function/7(cycles_cnt) -> Delay4/1, Compare To Constant/1
  Delay4/1 -> MATLAB Function/9("cycles_cnt ")
  Delay5/1 -> MATLAB Function/8("cnt_max_mat ")
  Delay6/1 -> MATLAB Function/7(e_old)
  Compare To Constant/1 -> Logical Operator/2
  Relational Operator/1 -> Logical Operator/1
  Constant/1 -> Relational Operator/2
  Rate Transition5/1 -> Delay6/1, Relational Operator/1
  Logical Operator/1 -> Stop Simulation/1
  Rate Transition6/1 -> To Workspace18/1, Delay5/1

== system AWES3_CL_wTether_v4_PM/Visualization ==
  AirframeOutput_Bus : Inport
  Ft : Inport  Port=2
  Bus Selector : BusSelector  OutputSignals=longlath,eta_OB_rad
  Clock : Clock
  Constant : Constant  Value=1500
  Demux : Demux  Outputs=3
  Display : Display
  MATLAB Function3 : MATLAB Function  TreatAsAtomicUnit=on
  Mux6 : Mux  Inputs=5
  Rate Transition2 : RateTransition  InitialCondition=zeros(9,1)  OutPortSampleTime=simInit.Ts_vis
  Selector : Selector  InputPortWidth=9  IndexOptions=Index vector (dialog)  Indices=9  OutputSizes=1
  Switch : Switch  Criteria=u2 > Threshold  Threshold=0.7  SaturateOnIntegerOverflow=off  InputSameDT=off
  Tether Rupture1 : Subsystem
  Tether Rupture2 : Subsystem
  To Workspace : ToWorkspace  Commented=on  VariableName=visualization_trim  SaveFormat=Timeseries  SampleTime=-1
  advanced_graphical_model : MATLABFcn  MATLABFcn=visualize_vehicle  OutputDimensions=0
  hold max : Subsystem
  wires:
  Demux/3 -> MATLAB Function3/3(z)
  Rate Transition2/1 -> Selector/1, advanced_graphical_model/1
  Bus Selector/1 -> Demux/1  "<longlath>"
  MATLAB Function3/1(y) -> Mux6/1
  Clock/1 -> Switch/2, Mux6/3
  Mux6/1 -> To Workspace/1, Rate Transition2/1
  Demux/1 -> MATLAB Function3/2(long)
  Demux/2 -> MATLAB Function3/1(lat)
  AirframeOutput_Bus/1 -> Bus Selector/1
  Bus Selector/2 -> Mux6/2  "<eta_OB_rad>"
  Switch/1 -> Mux6/4, hold max/1(In1)
  Constant/1 -> Switch/3
  Ft/1 -> Switch/1
  Selector/1 -> Tether Rupture1/1(In1)
  hold max/1(Out1) -> Tether Rupture2/1(In1), Display/1, Mux6/5

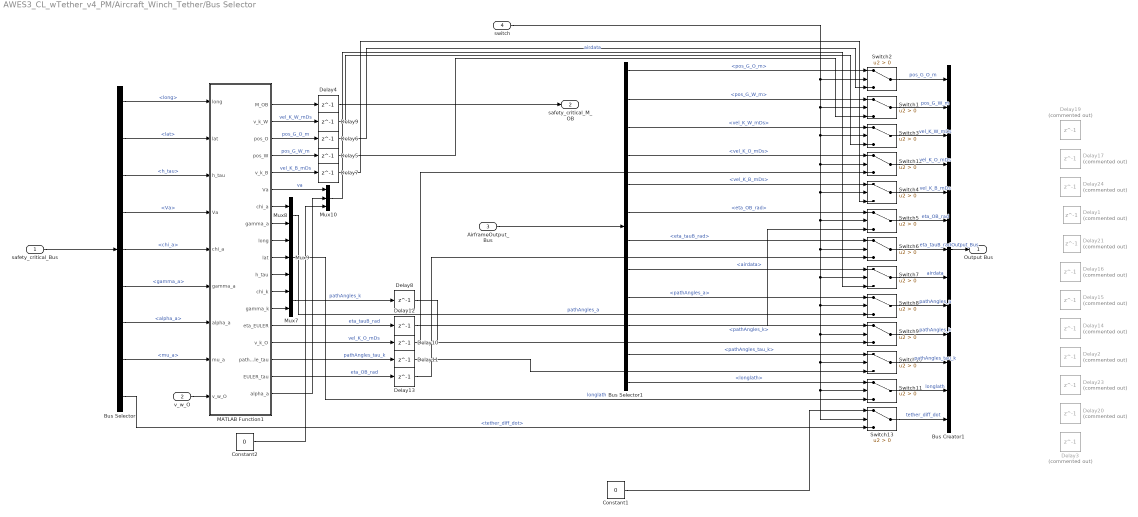
== system AWES3_CL_wTether_v4_PM/Aircraft_Winch_Tether/Bus Selector ==
  safety_critical_Bus : Inport
  v_w_O : Inport  Port=2
  AirframeOutput_Bus : Inport  Port=3
  switch : Inport  Port=4
  Bus Creator1 : BusCreator  Inputs=13
  Bus Selector : BusSelector  OutputSignals=long,lat,h_tau,Va,chi_a,gamma_a,alpha_a,mu_a,tether_diff_dot
  Bus Selector1 : BusSelector  OutputSignals=pos_G_O_m,pos_G_W_m,vel_K_W_mDs,vel_K_O_mDs,vel_K_B_mDs,eta_OB_rad,eta_tauB_rad,airdata,pathAngles_a,pathAngles_k,pathAngles_tau_k,longlath
  Constant1 : Constant  Value=0
  Constant2 : Constant  Value=0
  Delay1 : Delay  Commented=on  DelayLength=1  InitialCondition=simInit.v_k_O_init
  Delay10 : Delay  DelayLength=1  InitialCondition=simInit.v_k_O_init
  Delay11 : Delay  DelayLength=1  InitialCondition=zeros(2,1)
  Delay12 : Delay  DelayLength=1  InitialCondition=simInit.EULER_init
  Delay13 : Delay  DelayLength=1  InitialCondition=x0_sim(4:6)
  Delay14 : Delay  Commented=on  DelayLength=1  InitialCondition=x0_sim(1:3)
  Delay15 : Delay  Commented=on  DelayLength=1  InitialCondition=simInit.EULER_init
  Delay16 : Delay  Commented=on  DelayLength=1  InitialCondition=x0_sim(4:6)
  Delay17 : Delay  Commented=on  DelayLength=1  InitialCondition=simInit.pos_W_init
  Delay19 : Delay  Commented=on  DelayLength=1  InitialCondition=simInit.pos_O_init
  Delay2 : Delay  Commented=on  DelayLength=1  InitialCondition=simInit.pathangles_k_init'
  Delay20 : Delay  Commented=on  DelayLength=1  InitialCondition=zeros(2,1)
  Delay21 : Delay  Commented=on  DelayLength=1  InitialCondition=simInit.v_k_B_init
  Delay23 : Delay  Commented=on  DelayLength=1  InitialCondition=simInit.pathangles_k_init
  Delay24 : Delay  Commented=on  DelayLength=1  InitialCondition=simInit.v_k_W_init
  Delay3 : Delay  Commented=on  DelayLength=1  InitialCondition=x0_sim(10:12)
  Delay4 : Delay  DelayLength=1  InitialCondition=simInit.M_OB
  Delay5 : Delay  DelayLength=1  InitialCondition=simInit.pos_W_init
  Delay6 : Delay  DelayLength=1  InitialCondition=simInit.pos_O_init'
  Delay7 : Delay  DelayLength=1  InitialCondition=simInit.v_k_B_init
  Delay8 : Delay  DelayLength=1  InitialCondition=simInit.pathangles_k_init
  Delay9 : Delay  DelayLength=1  InitialCondition=simInit.v_k_W_init
  MATLAB Function1 : MATLAB Function  TreatAsAtomicUnit=on
  Mux10 : Mux  Inputs=3
  Mux7 : Mux  Inputs=2
  Mux8 : Mux  Inputs=2
  Mux9 : Mux  Inputs=3
  Switch{1..13} (13 alike) : Switch  Criteria=u2 > Threshold  SaturateOnIntegerOverflow=off  InputSameDT=off
  Output Bus : Outport
  safety_critical_M_OB : Outport  Port=2
  wires:
  MATLAB Function1/12(chi_k) -> Mux7/1
  MATLAB Function1/8(gamma_a) -> Mux8/2
  Constant2/1 -> Mux10/3
  MATLAB Function1/7(chi_a) -> Mux8/1
  Mux9/1 -> Switch11/3  "longlath"
  MATLAB Function1/10(lat) -> Mux9/2
  MATLAB Function1/13(gamma_k) -> Mux7/2
  MATLAB Function1/9(long) -> Mux9/1
  MATLAB Function1/6(Va) -> Mux10/1  "va"
  MATLAB Function1/11(h_tau) -> Mux9/3
  MATLAB Function1/18(alpha_a) -> Mux10/2
  safety_critical_Bus/1 -> Bus Selector/1
  Bus Selector/1 -> MATLAB Function1/1("long ")  "<long>"
  Bus Selector/2 -> MATLAB Function1/2("lat ")  "<lat>"
  Bus Selector/3 -> MATLAB Function1/3("h_tau ")  "<h_tau>"
  Bus Selector/4 -> MATLAB Function1/4("Va ")  "<Va>"
  Bus Selector/5 -> MATLAB Function1/5("chi_a ")  "<chi_a>"
  Bus Selector/6 -> MATLAB Function1/6("gamma_a ")  "<gamma_a>"
  switch/1 -> Switch12/2, Switch4/2, Switch6/2, Switch7/2, Switch8/2, Switch9/2, Switch10/2, Switch13/2, Switch11/2, Switch5/2, Switch3/2, Switch1/2, Switch2/2
  MATLAB Function1/3(pos_O) -> Delay6/1  "pos_G_O_m"
  MATLAB Function1/4(pos_W) -> Delay5/1  "pos_G_W_m"
  MATLAB Function1/2(v_k_W) -> Delay9/1  "vel_K_W_mDs"
  MATLAB Function1/15(v_k_O) -> Delay10/1  "vel_K_O_mDs"
  MATLAB Function1/5(v_k_B) -> Delay7/1  "vel_K_B_mDs"
  MATLAB Function1/17(EULER_tau) -> Delay13/1  "eta_OB_rad"
  Mux10/1 -> Switch7/3  "airdata"
  Mux8/1 -> Switch8/3  "pathAngles_a"
  Mux7/1 -> Delay8/1  "pathAngles_k"
  MATLAB Function1/16(pathangle_tau) -> Delay11/1  "pathAngles_tau_k"
  AirframeOutput_Bus/1 -> Bus Selector1/1
  Switch2/1 -> Bus Creator1/1  "pos_G_O_m"
  Switch1/1 -> Bus Creator1/2  "pos_G_W_m"
  Switch11/1 -> Bus Creator1/12  "longlath"
  Switch10/1 -> Bus Creator1/11  "pathAngles_tau_k"
  Switch9/1 -> Bus Creator1/10  "pathAngles_k"
  Switch8/1 -> Bus Creator1/9  "pathAngles_a"
  Switch7/1 -> Bus Creator1/8  "airdata"
  Switch6/1 -> Bus Creator1/7  "eta_tauB_rad"
  Switch5/1 -> Bus Creator1/6  "eta_OB_rad"
  Switch4/1 -> Bus Creator1/5  "vel_K_B_mDs"
  Switch12/1 -> Bus Creator1/4  "vel_K_O_mDs"
  Switch3/1 -> Bus Creator1/3  "vel_K_W_mDs"
  Bus Selector1/1 -> Switch2/1  "<pos_G_O_m>"
  Bus Selector1/2 -> Switch1/1  "<pos_G_W_m>"
  Bus Selector1/3 -> Switch3/1  "<vel_K_W_mDs>"
  Bus Selector1/4 -> Switch12/1  "<vel_K_O_mDs>"
  Bus Selector1/5 -> Switch4/1  "<vel_K_B_mDs>"
  Bus Selector1/6 -> Switch5/1  "<eta_OB_rad>"
  Bus Selector1/7 -> Switch6/1  "<eta_tauB_rad>"
  Bus Selector1/12 -> Switch11/1  "<longlath>"
  Bus Selector1/11 -> Switch10/1  "<pathAngles_tau_k>"
  Bus Selector1/10 -> Switch9/1  "<pathAngles_k>"
  Bus Selector1/9 -> Switch8/1  "<pathAngles_a>"
  Bus Selector1/8 -> Switch7/1  "<airdata>"
  v_w_O/1 -> MATLAB Function1/9(v_w_O)
  Bus Selector/8 -> MATLAB Function1/8(mu_a)  "<mu_a>"
  Bus Selector/7 -> MATLAB Function1/7("alpha_a ")  "<alpha_a>"
  Bus Creator1/1 -> Output Bus/1  "Output_Bus"
  MATLAB Function1/1(M_OB) -> Delay4/1
  MATLAB Function1/14(eta_EULER) -> Delay12/1  "eta_tauB_rad"
  Delay4/1 -> safety_critical_M_OB/1
  Bus Selector/9 -> Switch13/3  "<tether_diff_dot>"
  Switch13/1 -> Bus Creator1/13  "tether_diff_dot"
  Constant1/1 -> Switch13/1
  Delay5/1 -> Switch1/3
  Delay6/1 -> Switch2/3
  Delay7/1 -> Switch4/3
  Delay9/1 -> Switch3/3
  Delay8/1 -> Switch9/3
  Delay10/1 -> Switch12/3
  Delay11/1 -> Switch10/3
  Delay12/1 -> Switch5/3
  Delay13/1 -> Switch6/3

== system AWES3_CL_wTether_v4_PM/Aircraft_Winch_Tether/ForcesAndMoments1 ==
  Ft_G_W : Inport
  Ft_tot : Inport  Port=2
  complex_tether : Inport  Port=3
  airdata : Inport  Port=4  PortDimensions=[3,1]
  pos_W : Inport  Port=5
  M_OB : Inport  Port=6  PortDimensions=[3,3]
  Constant : Constant  Value=0
  Constant1 : Constant  Value=u0_sim
  MATLAB Function : MATLAB Function  TreatAsAtomicUnit=on
  Sum : Sum  Inputs=|++
  Sum1 : Sum  Inputs=|++
  Switch : Switch  Criteria=u2 > Threshold  SaturateOnIntegerOverflow=off  InputSameDT=off
  Terminator : Terminator
  Terminator2 : Terminator
  TetherDragApprox : MATLAB Function  TreatAsAtomicUnit=on
  allForcesTorques_exceptAero : MATLAB Function  TreatAsAtomicUnit=on
  F_tot_A : Outport  VectorParamsAs1DForOutWhenUnconnected=off
  F_a_B : Outport  Port=2  VectorParamsAs1DForOutWhenUnconnected=off
  tag scope: F_a_A=global
  wires:
  allForcesTorques_exceptAero/1(F_A) -> Sum1/1  "F_A"
  Ft_G_W/1 -> allForcesTorques_exceptAero/2(F_t_W)
  MATLAB Function/1(F_a_A) -> Sum1/2, [F_a_A]  "F_a_B"
  Sum1/1 -> Sum/1
  M_OB/1 -> allForcesTorques_exceptAero/1(DCM), TetherDragApprox/3(M_OB)
  airdata/1 -> TetherDragApprox/1(airdata), MATLAB Function/1(airdata), allForcesTorques_exceptAero/3(airdata)
  Sum/1 -> F_tot_A/1
  TetherDragApprox/2(Ftd_A2) -> Switch/3
  TetherDragApprox/1(Ftd_A) -> Terminator/1
  pos_W/1 -> allForcesTorques_exceptAero/4(pos_W), TetherDragApprox/2(pos_W)
  MATLAB Function/2(F_a_B) -> F_a_B/1
  Ft_tot/1 -> allForcesTorques_exceptAero/5(F_t_tot)
  Switch/1 -> Sum/2
  complex_tether/1 -> allForcesTorques_exceptAero/6(Ft_flag), Switch/2
  Constant/1 -> Switch/1
  Constant1/1 -> MATLAB Function/2(u_trim)
  allForcesTorques_exceptAero/2(Ftot) -> Terminator2/1

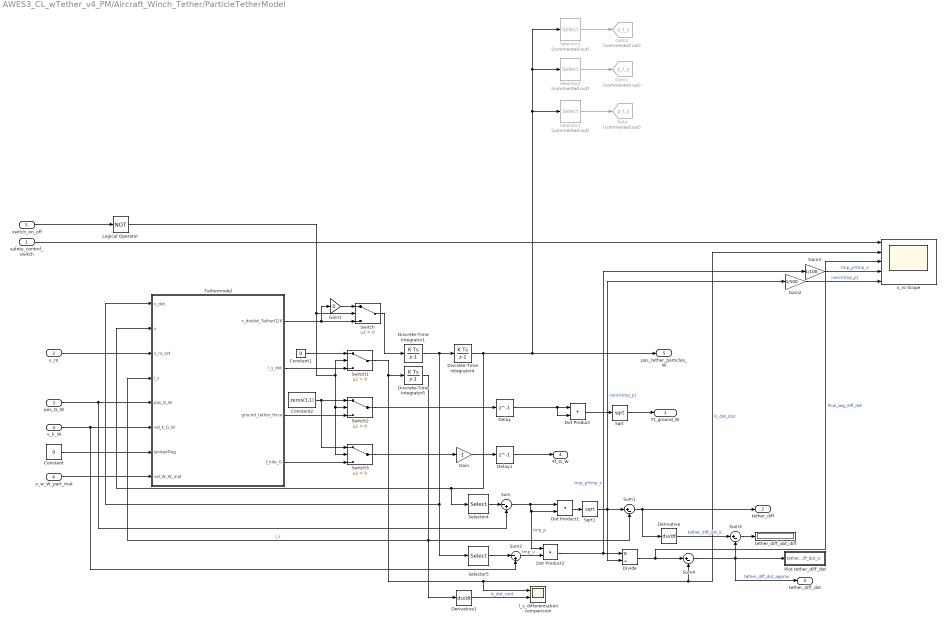
== system AWES3_CL_wTether_v4_PM/Aircraft_Winch_Tether/ParticleTetherModel ==
  safety_control_switch : Inport
  v_ro : Inport  Port=2
  pos_G_W : Inport  Port=3
  v_k_W : Inport  Port=4
  switch_on_off : Inport  Port=5
  v_w_W_part_mat : Inport  Port=6
  Constant : Constant  Value=0
  Constant1 : Constant  Value=0
  Constant2 : Constant  Value=zeros(3,1)
  Delay : Delay  DelayLength=1  InitialCondition=zeros(3,1)
  Delay1 : Delay  DelayLength=1  InitialCondition=zeros(3,1)
  Derivative : Derivative
  Derivative1 : Derivative
  Discrete-Time Integrator1 : DiscreteIntegrator  InitialCondition=simInit.vel_p_init  SampleTime=simInit.dt  ICPrevOutput=DiscIntNeverNeededParam  ICPrevScaledInput=DiscIntNeverNeededParam
  Discrete-Time Integrator4 : DiscreteIntegrator  InitialCondition=simInit.pos_p_init -1  SampleTime=simInit.dt  LowerSaturationLimit=0  ICPrevOutput=DiscIntNeverNeededParam  ICPrevScaledInput=DiscIntNeverNeededParam
  Discrete-Time Integrator5 : DiscreteIntegrator  InitialCondition=T.l0  SampleTime=simInit.dt  ICPrevOutput=DiscIntNeverNeededParam  ICPrevScaledInput=DiscIntNeverNeededParam
  Divide : Product  Inputs=*/
  Dot Product : DotProduct  OutDataTypeStr=Inherit: Inherit via internal rule
  Dot Product1 : DotProduct  OutDataTypeStr=Inherit: Inherit via internal rule
  Dot Product2 : DotProduct  OutDataTypeStr=Inherit: Inherit via internal rule
  Gain : Gain  Gain=-1
  Gain1 : Gain  Gain=0
  Gain2 : Gain  Gain=1/100
  Gain3 : Gain  Gain=1/100
  Goto : Goto  Commented=on  GotoTag=p_t_z  TagVisibility=global
  Goto1 : Goto  Commented=on  GotoTag=p_t_y  TagVisibility=global
  Goto2 : Goto  Commented=on  GotoTag=p_t_x  TagVisibility=global
  Logical Operator : Logic  Operator=NOT  AllPortsSameDT=off  OutDataTypeStr=boolean
  Plot tether_diff_dot : Subsystem
  Selector1 : Selector  Commented=on  InputPortWidth=3*T.np  IndexOptions=Index vector (dialog)  Indices=3:3:3*T.np  OutputSizes=1
  Selector2 : Selector  Commented=on  InputPortWidth=3*T.np  IndexOptions=Index vector (dialog)  Indices=2:3:3*T.np-1  OutputSizes=1
  Selector3 : Selector  Commented=on  InputPortWidth=3*T.np  IndexOptions=Index vector (dialog)  Indices=1:3:3*T.np-2  OutputSizes=1
  Selector4 : Selector  InputPortWidth=15  IndexOptions=Index vector (dialog)  Indices=[13 14 15]  OutputSizes=3
  Selector5 : Selector  InputPortWidth=15  IndexOptions=Index vector (dialog)  Indices=[13 14 15]  OutputSizes=3
  Sqrt : Sqrt
  Sqrt1 : Sqrt
  Sum : Sum  Inputs=|-+
  Sum1 : Sum  Inputs=|+-
  Sum2 : Sum  Inputs=|-+
  Sum3 : Sum  Inputs=|+-
  Sum4 : Sum  Inputs=|+-
  Switch{,1..3} (4 alike) : Switch  Criteria=u2 > Threshold  SaturateOnIntegerOverflow=off  InputSameDT=off
  Tethermodel : MATLAB Function  TreatAsAtomicUnit=on
  l_s_differentiation comparision : Scope  NumInputPorts=2
  tether_diff_dot_diff : Display
  v_ro Scope : Scope  NumInputPorts=5
  Ft_ground_W : Outport  VectorParamsAs1DForOutWhenUnconnected=off
  tether_diff : Outport  Port=2
  tether_diff_dot : Outport  Port=3
  Ft_G_W : Outport  Port=4  VectorParamsAs1DForOutWhenUnconnected=off
  pos_tether_particles_W : Outport  Port=5  VectorParamsAs1DForOutWhenUnconnected=off
  wires:
  Switch2/1 -> Delay/1
  Switch3/1 -> Gain/1
  Tethermodel/1(x_dotdot_TetherG2K) -> Gain1/1, Switch/3
  Gain/1 -> Delay1/1
  v_w_W_part_mat/1 -> Tethermodel/8(vel_W_W_mat)
  v_ro/1 -> Tethermodel/3(v_ro_set)
  Constant/1 -> Tethermodel/7(landedFlag)
  Discrete-Time Integrator1/1 -> Selector5/1, Tethermodel/1(x_dot), Discrete-Time Integrator4/1
  switch_on_off/1 -> Logical Operator/1
  Constant1/1 -> Switch1/1
  Switch/1 -> Discrete-Time Integrator1/1
  Switch1/1 -> Discrete-Time Integrator5/1, l_s_differentiation comparision/1, Sum4/2, v_ro Scope/2  "ls_dot_disc"
  Constant2/1 -> Switch3/1, Switch2/1
  Tethermodel/3(ground_tether_force) -> Switch2/3
  Tethermodel/4(f_kite_G) -> Switch3/3
  Gain1/1 -> Switch/1
  Delay/1 -> Dot Product/2, Dot Product/1
  Selector3/1 -> Goto2/1
  Selector1/1 -> Goto/1
  Selector2/1 -> Goto1/1
  Dot Product/1 -> Sqrt/1
  Sqrt/1 -> Ft_ground_W/1
  Discrete-Time Integrator4/1 -> Selector3/1, Selector2/1, Selector1/1, pos_tether_particles_W/1, Selector4/1, Tethermodel/2(x)
  Logical Operator/1 -> Switch2/2, Switch3/2, Switch1/2, Switch/2
  Delay1/1 -> Ft_G_W/1
  Selector4/1 -> Sum/1
  Sum/1 -> Dot Product2/1, Dot Product1/2, Dot Product1/1  "tmp_p"
  Dot Product1/1 -> Sqrt1/1
  Sqrt1/1 -> Divide/2, Gain2/1, Sum1/1  "norm(tmp_p)"
  Sum1/1 -> Derivative/1, tether_diff/1
  Derivative/1 -> Sum3/1  "tether_diff_dot_is"
  Selector5/1 -> Sum2/1
  Sum2/1 -> Dot Product2/2  "tmp_v"
  Dot Product2/1 -> Gain3/1, Divide/1  "tmp_p*tmp_v"
  pos_G_W/1 -> Tethermodel/5(pos_G_W), Sum/2
  v_k_W/1 -> Tethermodel/6(vel_k_G_W), Sum2/2
  Divide/1 -> v_ro Scope/3, Sum4/1  "final_seg_diff_dot"
  Tethermodel/2(l_s_dot) -> Switch1/3
  Sum4/1 -> tether_diff_dot/1, Plot tether_diff_dot/1(tether_diff_dot_is), Sum3/2  "tether_diff_dot_approx"
  Sum3/1 -> tether_diff_dot_diff/1
  safety_control_switch/1 -> v_ro Scope/1
  Discrete-Time Integrator5/1 -> Derivative1/1, Tethermodel/4(l_s), Sum1/2  "l_s"
  Derivative1/1 -> l_s_differentiation comparision/2  "ls_dot_cont"
  Gain2/1 -> v_ro Scope/5  "norm(tmp_p)"
  Gain3/1 -> v_ro Scope/4  "tmp_p*tmp_v"

== system AWES3_CL_wTether_v4_PM/Aircraft_Winch_Tether/Subsystem ==
  alpha_a_c : Inport
  mu_a_c : Inport  Port=2
  v_w_O : Inport  Port=3
  F_a_A : Inport  Port=4
  6DoFKinematics1 : Subsystem
  Bus Creator : BusCreator  Inputs=12
  Demux : Demux  Outputs=3
  Mux : Mux  Inputs=3
  Output_Bus : Outport
  M_OB : Outport  Port=2
  wires:
  mu_a_c/1 -> 6DoFKinematics1/3(mu_a_c)
  6DoFKinematics1/1(M_OB) -> M_OB/1
  F_a_A/1 -> 6DoFKinematics1/1(F_a_A)
  6DoFKinematics1/2(pos_O) -> Bus Creator/1  "pos_G_O_m"
  Demux/2 -> Mux/3
  6DoFKinematics1/6(v_k_B) -> Bus Creator/5  "vel_K_B_mDs"
  v_w_O/1 -> 6DoFKinematics1/4(v_w_O)
  6DoFKinematics1/8(phi,theta,psi_tau) -> Bus Creator/7  "eta_tauB_rad"
  6DoFKinematics1/13(pos_S) -> Bus Creator/12  "longlath"
  6DoFKinematics1/4(v_k_W) -> Bus Creator/3  "vel_K_W_mDs"
  Mux/1 -> Bus Creator/8  "airdata"
  alpha_a_c/1 -> 6DoFKinematics1/2(alpha_a_c)
  6DoFKinematics1/7(phi,theta,psi) -> Bus Creator/6  "eta_OB_rad"
  6DoFKinematics1/10(pathangles_a) -> Bus Creator/9  "pathAngles_a"
  6DoFKinematics1/11(pathangles_k) -> Bus Creator/10  "pathAngles_k"
  6DoFKinematics1/5(v_k_O) -> Bus Creator/4  "vel_K_O_mDs"
  Demux/3 -> Mux/2
  Demux/1 -> Mux/1  "va"
  6DoFKinematics1/12(pathangle_tau) -> Bus Creator/11  "pathAngles_tau_k"
  6DoFKinematics1/9(x_A) -> Demux/1
  6DoFKinematics1/3(pos_W) -> Bus Creator/2  "pos_G_W_m"
  Bus Creator/1 -> Output_Bus/1  "Output_Bus"
